simulink model "Task_1C"  (R2022a)
settings: Solver=VariableStepAuto  StartTime=0.0  StopTime=50  RelTol=1e-3
values from neighbouring files (symbols this model uses):
  K = 1    [Parameter_Setup.m]
  La = 0.001    [Parameter_Setup.m]
  N = 1    [Parameter_Setup.m]
  Ra = 1    [Parameter_Setup.m]
settings Model: Creator=jpcas  LastModifiedBy=jpcas

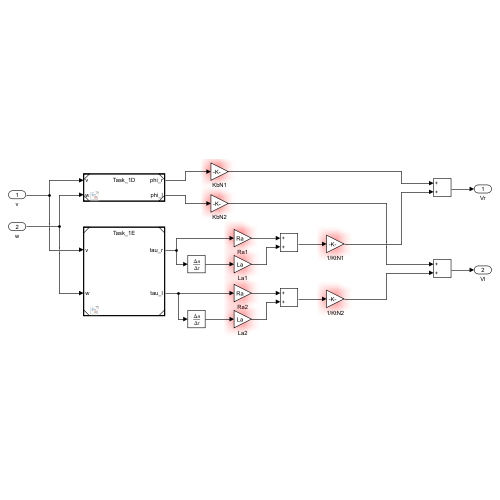
[thumbnail: Simulink's stored preview of the top-level diagram]
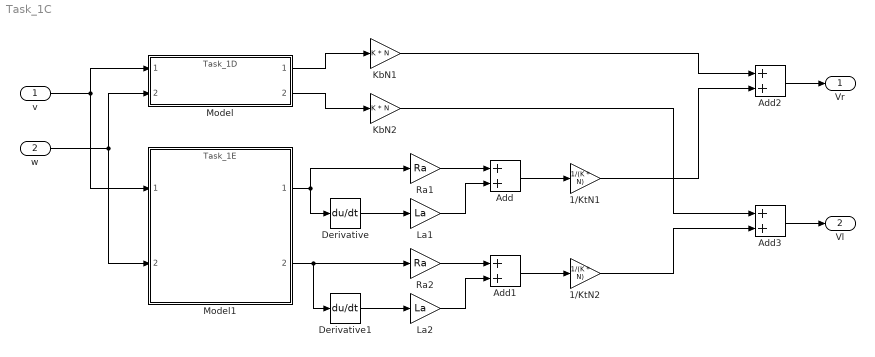
== system Task_1C ==
  v : Inport
  w : Inport  Port=2
  1/KtN1 : Gain  Gain=1/(K * N)
  1/KtN2 : Gain  Gain=1/(K * N)
  Add{,1..3} (4 alike) : Sum
  Derivative : Derivative
  Derivative1 : Derivative
  KbN1 : Gain  Gain=K * N
  KbN2 : Gain  Gain=K * N
  La1 : Gain  Gain=La
  La2 : Gain  Gain=La
  Model : ModelReference  ModelNameDialog=Task_1D  SimulationMode=Normal  ModelReferenceVersion=1.4
  Model1 : ModelReference  ModelNameDialog=Task_1E  SimulationMode=Normal  ModelReferenceVersion=1.3
  Ra1 : Gain  Gain=Ra
  Ra2 : Gain  Gain=Ra
  Vr : Outport
  Vl : Outport  Port=2
  wires:
  v/1 -> Model/1, Model1/1
  w/1 -> Model1/2, Model/2
  Model/2 -> KbN2/1
  Model/1 -> KbN1/1
  Model1/1 -> Ra1/1, Derivative/1
  Ra1/1 -> Add/1
  La1/1 -> Add/2
  Derivative/1 -> La1/1
  Model1/2 -> Derivative1/1, Ra2/1
  La2/1 -> Add1/2
  Ra2/1 -> Add1/1
  Derivative1/1 -> La2/1
  Add1/1 -> 1/KtN2/1
  Add/1 -> 1/KtN1/1
  1/KtN2/1 -> Add3/2
  KbN2/1 -> Add3/1
  KbN1/1 -> Add2/1
  1/KtN1/1 -> Add2/2
  Add3/1 -> Vl/1
  Add2/1 -> Vr/1
